simulink model "system2"  (R2023b)
settings: Solver=VariableStepAuto  StartTime=0.0  StopTime=10.0  RelTol=1e-3
undefined symbols (not defined in the file): c, g, l, m, x0
settings Model: Creator=roman  LastModifiedBy=roman

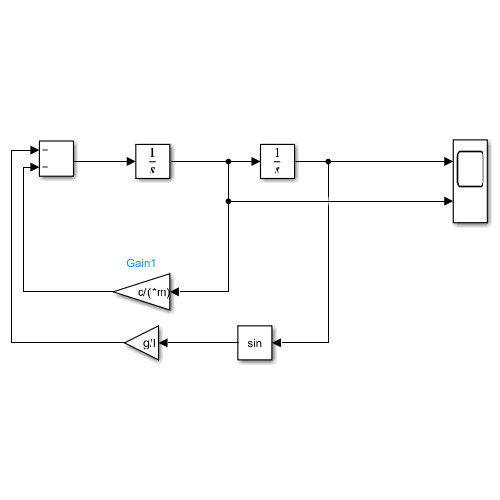
[thumbnail: Simulink's stored preview of the top-level diagram]
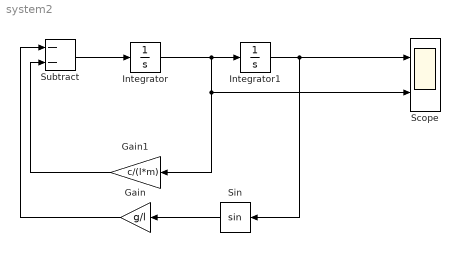
== system system2 ==
  Gain : Gain  Gain=g/l
  Gain1 : Gain  Gain=c/(l*m)
  Integrator : Integrator  InitialCondition=x0(2)
  Integrator1 : Integrator  InitialCondition=x0(1)
  Scope : Scope  NumInputPorts=2
  Sin : Trigonometry
  Subtract : Sum  Inputs=--
  wires:
  Integrator/1 -> Gain1/1, Scope/2, Integrator1/1
  Subtract/1 -> Integrator/1
  Integrator1/1 -> Sin/1, Scope/1
  Sin/1 -> Gain/1
  Gain/1 -> Subtract/1
  Gain1/1 -> Subtract/2
